simulink model "ptransform3TO2"  (R2021a)
settings: Solver=VariableStepAuto  StartTime=0.0  StopTime=1  RelTol=1e-3
libraries: spsPLL3phLib x1, spsabctoAlphaBetaZeroLib x1, spsabctodq0Lib x1
settings Model: Creator=User  LastModifiedBy=User

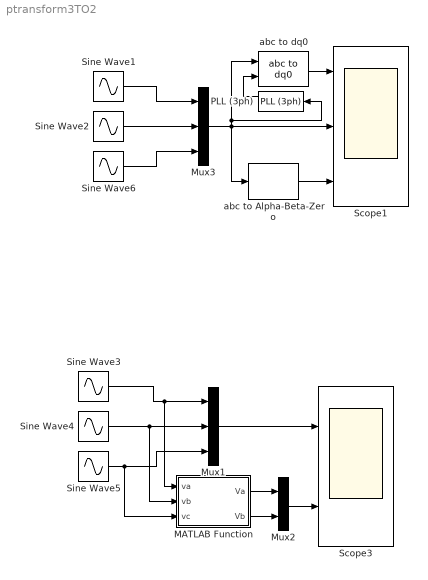
== system ptransform3TO2 ==
  MATLAB Function : MATLAB Function  TreatAsAtomicUnit=on
  Mux1 : Mux  Inputs=3
  Mux2 : Mux  Inputs=2
  Mux3 : Mux  Inputs=3
  PLL (3ph) : spsPLL3phLib/PLL (3ph)  Fmin=45  Par_Init=[0, 50]  ParK=[180, 3200, 1]  TcD=1e-4  MaxRateChangeFreq=12  FilterCutOffFreq=25  Ts=0  AGC=on
  Scope1 : Scope  NumInputPorts=3
  Scope3 : Scope  NumInputPorts=2
  Sine Wave1 : Sin  Frequency=50*2*pi  SampleTime=0.0001
  Sine Wave2 : Sin  Frequency=50*2*pi  Phase=-2*pi/3  SampleTime=.0001
  Sine Wave3 : Sin  Frequency=50*2*pi  SampleTime=0.0001
  Sine Wave4 : Sin  Frequency=50*2*pi  Phase=-2*pi/3  SampleTime=.0001
  Sine Wave5 : Sin  Frequency=50*2*pi  Phase=2*pi/3  SampleTime=.0001
  Sine Wave6 : Sin  Frequency=50*2*pi  Phase=2*pi/3  SampleTime=.0001
  abc to Alpha-Beta-Zero : spsabctoAlphaBetaZeroLib/abc to Alpha-Beta-Zero
      settings: SourceProductBaseCode=PS
  abc to dq0 : spsabctodq0Lib/abc to dq0  Alignment=90 degrees behind phase A axis
  wires:
  Sine Wave5/1 -> MATLAB Function/3(vc), Mux1/3
  Sine Wave4/1 -> MATLAB Function/2(vb), Mux1/2
  Sine Wave3/1 -> MATLAB Function/1(va), Mux1/1
  Mux1/1 -> Scope3/1
  MATLAB Function/1(Va) -> Mux2/1
  MATLAB Function/2(Vb) -> Mux2/2
  Mux2/1 -> Scope3/2
  abc to Alpha-Beta-Zero/1 -> Scope1/3
  Mux3/1 -> PLL (3ph)/1, abc to dq0/1, abc to Alpha-Beta-Zero/1, Scope1/2
  Sine Wave6/1 -> Mux3/3
  Sine Wave2/1 -> Mux3/2
  Sine Wave1/1 -> Mux3/1
  abc to dq0/1 -> Scope1/1
  PLL (3ph)/2 -> abc to dq0/2

== matlab function ptransform3TO2/MATLAB Function ==
  data: va input; Va output; vb input; vc input; Vb output
function [Va,Vb] = fcn(va,vb,vc)
Va = va - .5*vb - .5*vc
Vb = -(sqrt(3)/2)*vb + (sqrt(3)/2)*vc
end
